simulink model "sliding_quadcopter"  (Simulink 7.9)
settings: Solver=ode4  StartTime=0.0  StopTime=t_end  FixedStep=.01  RelTol=1e-3
values from neighbouring files (symbols this model uses):
  C = [0 0 0]    [gen_smc_starter.m]    (also in pid_starter.m; sliding_starter.m)
  CC_nom = diag([C_nom,Cd_nom])    [gen_smc_starter.m]    (also in sliding_starter.m)
  Cd = [0 0 0]    [gen_smc_starter.m]    (also in pid_starter.m; sliding_starter.m)
  eta = [1 1 1 1]'    [gen_smc_starter.m]    (also in sliding_starter.m = [1 1 1 1 1 1]')
  g = 9.81    [gen_smc_starter.m]    (also in pid_starter.m; sliding_starter.m)
  H_nom = diag([m_nom,m_nom,m_nom,Ix_nom,Iy_nom,Iz_nom])    [gen_smc_starter.m]    (also in sliding_starter.m)
  I = [Ix Iy Iz]    [gen_smc_starter.m]    (also in pid_starter.m; sliding_starter.m)
  Kf = 100    [gen_smc_starter.m]    (also in pid_starter.m; sliding_starter.m)
  Km = 1    [gen_smc_starter.m]    (also in pid_starter.m; sliding_starter.m)
  l = .25    (= 0.25)    [gen_smc_starter.m]    (also in pid_starter.m; sliding_starter.m)
  lamb = [1 20 20 1]    [gen_smc_starter.m]    (also in sliding_starter.m = [5 100 5 .1 .1 .1])
  m = .5    (= 0.5)    [gen_smc_starter.m]    (also in pid_starter.m; sliding_starter.m)
  PSI = [.01 .0005 .0005 .001]'    [gen_smc_starter.m]    (also in sliding_starter.m = [.005 .005 .005 .005 .005 .005]')
  ref = [.1 0 .2 0 0 0]    [gen_smc_starter.m]    (also in pid_starter.m = [.1 -.1 .5 0 0 0]; sliding_starter.m = [0 2 1 0 0 0])
  step_time = [0 0 0]    [gen_smc_starter.m]    (also in pid_starter.m; sliding_starter.m)
  x0 = [0 0        0 0        .2 0        0 0        0 0        0 0        ]    [gen_smc_starter.m]    (also in pid_starter.m = [0 0        0 0        .1 0        0 0        0 0        0 0; sliding_starter.m = [0 0        0 0        .1 0        0 0        0 0        0 0)
settings Model: Creator=dwai  LastModifiedBy=dwai
settings DataIOCC: LimitDataPoints=off
settings DebuggingCC: AlgebraicLoopMsg=none

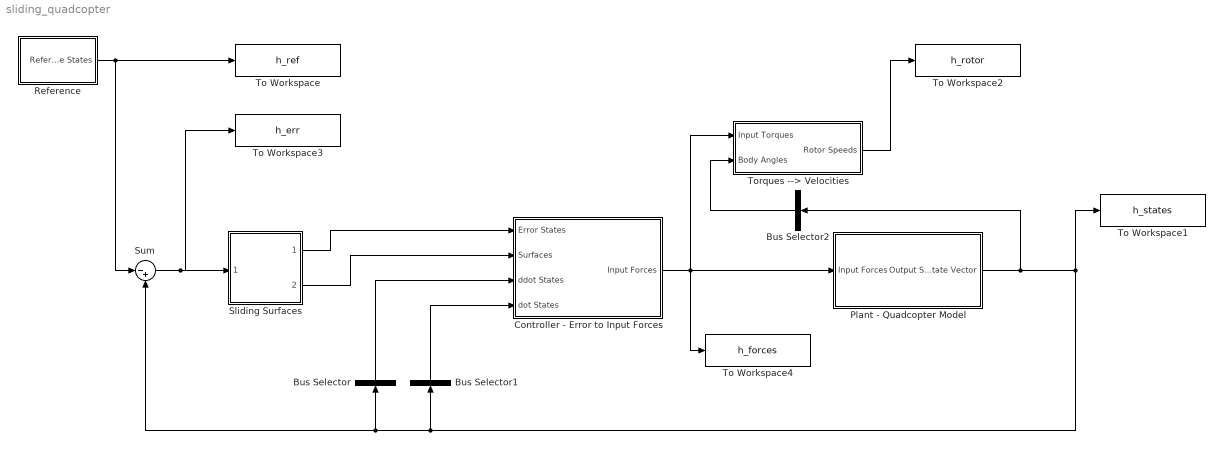
== system sliding_quadcopter ==
  Bus Selector : BusSelector  OutputSignals=x ddot,y ddot,z ddot,phi ddot,th ddot,psi ddot  OutputAsBus=on
  Bus Selector1 : BusSelector  OutputSignals=x dot,y dot,z dot,phi dot,th dot,psi dot  OutputAsBus=on
  Bus Selector2 : BusSelector  OutputSignals=phi,th,psi  OutputAsBus=on
  Controller - Error to Input Forces : Subsystem
  Plant - Quadcopter Model : Subsystem
  Reference : Subsystem
  Sliding Surfaces : Subsystem
  Sum : Sum  Inputs=|-+
  To Workspace : ToWorkspace  VariableName=h_ref  SampleTime=-1  SaveFormat=Timeseries
  To Workspace1 : ToWorkspace  VariableName=h_states  SampleTime=-1  SaveFormat=Timeseries
  To Workspace2 : ToWorkspace  VariableName=h_rotor  SampleTime=-1  SaveFormat=Timeseries
  To Workspace3 : ToWorkspace  VariableName=h_err  SampleTime=-1  SaveFormat=Timeseries
  To Workspace4 : ToWorkspace  VariableName=h_forces  SampleTime=-1  SaveFormat=Timeseries
  Torques --> Velocities : Subsystem
  wires:
  Plant - Quadcopter Model/1(Output State Vector) -> To Workspace1/1, Sum/2, Bus Selector/1, Bus Selector1/1, Bus Selector2/1
  Reference/1(Reference States) -> To Workspace/1, Sum/1
  Sum/1 -> To Workspace3/1, Sliding Surfaces/1(Error States)
  Sliding Surfaces/1(Err States) -> Controller - Error to Input Forces/1(Error States)
  Sliding Surfaces/2(Surfaces) -> Controller - Error to Input Forces/2(Surfaces)
  Bus Selector/1 -> Controller - Error to Input Forces/3(ddot States)
  Bus Selector1/1 -> Controller - Error to Input Forces/4(dot States)
  Controller - Error to Input Forces/1(Input Forces) -> Plant - Quadcopter Model/1(Input Forces), Torques --> Velocities/1(Input Torques), To Workspace4/1
  Torques --> Velocities/1(Rotor Speeds) -> To Workspace2/1
  Bus Selector2/1 -> Torques --> Velocities/2(Body Angles)

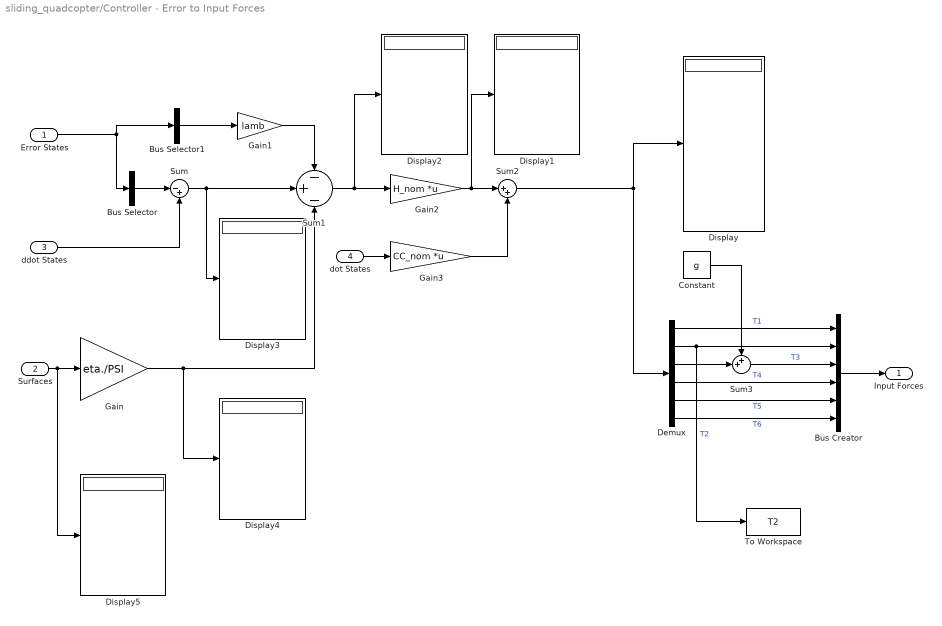
== system sliding_quadcopter/Controller - Error to Input Forces ==
  Error States : Inport
  Surfaces : Inport  Port=2
  ddot States : Inport  Port=3
  dot States : Inport  Port=4
  Bus Creator : BusCreator  Inputs=6
  Bus Selector : BusSelector  OutputSignals=xddot_err,yddot_err,zddot_err,phiddot_err,thddot_err,psiddot_err  OutputAsBus=on
  Bus Selector1 : BusSelector  OutputSignals=xdot_err,ydot_err,zdot_err,phidot_err,thdot_err,psidot_err  OutputAsBus=on
  Constant : Constant  Value=g
  Demux : Demux  Outputs=6
  Display{,1..5} (6 alike) : Display
  Gain : Gain  Gain=eta./PSI
  Gain1 : Gain  Gain=lamb
  Gain2 : Gain  Gain=H_nom  Multiplication=Matrix(K*u)
  Gain3 : Gain  Gain=CC_nom  Multiplication=Matrix(K*u)
  Sum : Sum  Inputs=|-+
  Sum1 : Sum  Inputs=-+-
  Sum2 : Sum  Inputs=|++
  Sum3 : Sum  Inputs=++|
  To Workspace : ToWorkspace  VariableName=T2  SampleTime=-1  SaveFormat=Timeseries
  Input Forces : Outport
  wires:
  Error States/1 -> Bus Selector/1, Bus Selector1/1
  Bus Creator/1 -> Input Forces/1
  Surfaces/1 -> Gain/1, Display5/1
  ddot States/1 -> Sum/2
  Bus Selector/1 -> Sum/1
  Bus Selector1/1 -> Gain1/1
  Gain/1 -> Sum1/3, Display4/1
  Sum/1 -> Sum1/2, Display3/1
  Gain1/1 -> Sum1/1
  dot States/1 -> Gain3/1
  Sum1/1 -> Gain2/1, Display2/1
  Gain2/1 -> Sum2/1, Display1/1
  Gain3/1 -> Sum2/2
  Sum2/1 -> Demux/1, Display/1
  Demux/1 -> Bus Creator/1  "T1"
  Demux/2 -> Bus Creator/2, To Workspace/1  "T2"
  Demux/4 -> Bus Creator/4  "T4"
  Demux/3 -> Sum3/2
  Sum3/1 -> Bus Creator/3  "T3"
  Constant/1 -> Sum3/1
  Demux/5 -> Bus Creator/5  "T5"
  Demux/6 -> Bus Creator/6  "T6"

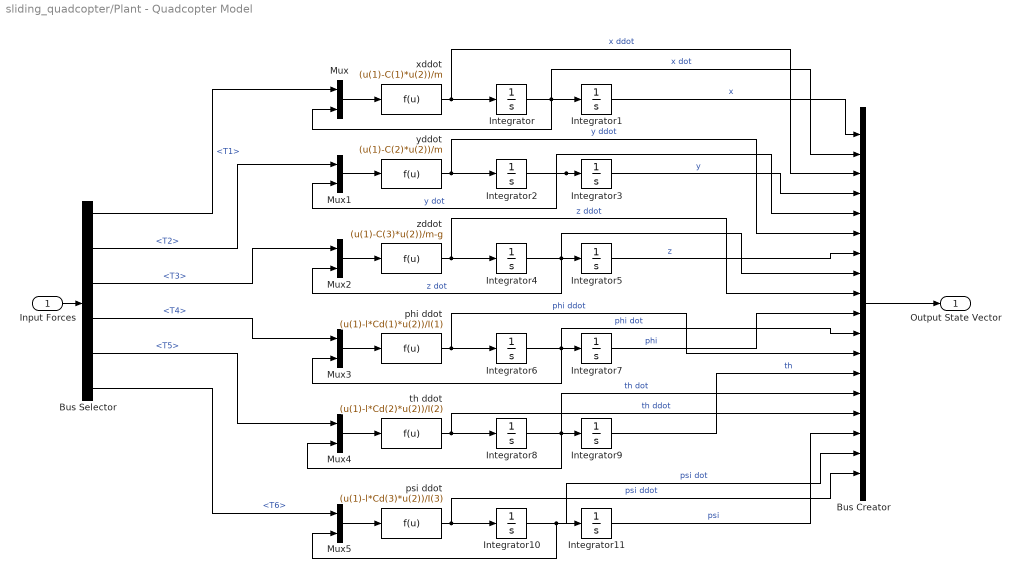
== system sliding_quadcopter/Plant - Quadcopter Model ==
  Input Forces : Inport
  Bus Creator : BusCreator  Inputs=18
  Bus Selector : BusSelector  OutputSignals=T1,T2,T3,T4,T5,T6
  Integrator : Integrator  InitialCondition=x0(2)
  Integrator1 : Integrator  InitialCondition=x0(1)
  Integrator10 : Integrator  InitialCondition=x0(12)
  Integrator11 : Integrator  InitialCondition=x0(11)
  Integrator2 : Integrator  InitialCondition=x0(4)
  Integrator3 : Integrator  InitialCondition=x0(3)
  Integrator4 : Integrator  InitialCondition=x0(6)
  Integrator5 : Integrator  InitialCondition=x0(5)
  Integrator6 : Integrator  InitialCondition=x0(8)
  Integrator7 : Integrator  InitialCondition=x0(7)
  Integrator8 : Integrator  InitialCondition=x0(10)
  Integrator9 : Integrator  InitialCondition=x0(9)
  Mux{,1..5} (6 alike) : Mux  Inputs=2
  phi ddot : Fcn  Expr=(u(1)-l*Cd(1)*u(2))/I(1)
  psi ddot : Fcn  Expr=(u(1)-l*Cd(3)*u(2))/I(3)
  th ddot : Fcn  Expr=(u(1)-l*Cd(2)*u(2))/I(2)
  xddot : Fcn  Expr=(u(1)-C(1)*u(2))/m
  yddot : Fcn  Expr=(u(1)-C(2)*u(2))/m
  zddot : Fcn  Expr=(u(1)-C(3)*u(2))/m-g
  Output State Vector : Outport
  wires:
  Bus Selector/6 -> Mux5/1  "<T6>"
  Bus Selector/5 -> Mux4/1  "<T5>"
  Bus Selector/4 -> Mux3/1  "<T4>"
  Bus Selector/3 -> Mux2/1  "<T3>"
  Bus Selector/2 -> Mux1/1  "<T2>"
  Bus Selector/1 -> Mux/1  "<T1>"
  Integrator11/1 -> Bus Creator/16  "psi"
  Integrator9/1 -> Bus Creator/13  "th"
  Integrator7/1 -> Bus Creator/10  "phi"
  Integrator5/1 -> Bus Creator/7  "z"
  Integrator3/1 -> Bus Creator/4  "y"
  Integrator1/1 -> Bus Creator/1  "x"
  Integrator10/1 -> Integrator11/1, Mux5/2, Bus Creator/17  "psi dot"
  psi ddot/1 -> Integrator10/1, Bus Creator/18  "psi ddot"
  Mux5/1 -> psi ddot/1
  Integrator8/1 -> Integrator9/1, Mux4/2, Bus Creator/14  "th dot"
  th ddot/1 -> Integrator8/1, Bus Creator/15  "th ddot"
  Mux4/1 -> th ddot/1
  Integrator6/1 -> Integrator7/1, Mux3/2, Bus Creator/11  "phi dot"
  phi ddot/1 -> Integrator6/1, Bus Creator/12  "phi ddot"
  Mux3/1 -> phi ddot/1
  Integrator4/1 -> Integrator5/1, Mux2/2, Bus Creator/8  "z dot"
  zddot/1 -> Integrator4/1, Bus Creator/9  "z ddot"
  Mux2/1 -> zddot/1
  Integrator2/1 -> Integrator3/1, Mux1/2, Bus Creator/5  "y dot"
  yddot/1 -> Integrator2/1, Bus Creator/6  "y ddot"
  Mux1/1 -> yddot/1
  Integrator/1 -> Integrator1/1, Mux/2, Bus Creator/2  "x dot"
  xddot/1 -> Integrator/1, Bus Creator/3  "x ddot"
  Mux/1 -> xddot/1
  Bus Creator/1 -> Output State Vector/1
  Input Forces/1 -> Bus Selector/1

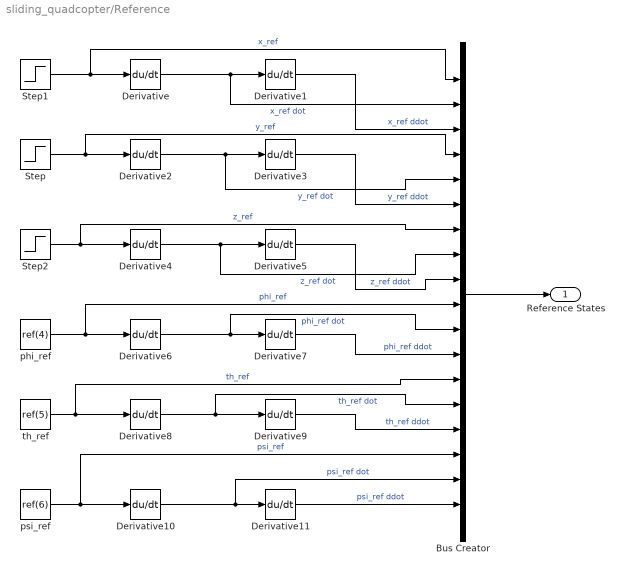
== system sliding_quadcopter/Reference ==
  Bus Creator : BusCreator  Inputs=18
  Derivative{,1..11} (12 alike) : Derivative
  Step : Step  Time=step_time(2)  After=ref(2)  SampleTime=0
  Step1 : Step  Time=step_time(1)  After=ref(1)  SampleTime=0
  Step2 : Step  Time=step_time(3)  After=ref(3)  SampleTime=0
  phi_ref : Constant  Value=ref(4)
  psi_ref : Constant  Value=ref(6)
  th_ref : Constant  Value=ref(5)
  Reference States : Outport
  wires:
  Derivative/1 -> Derivative1/1, Bus Creator/2  "x_ref dot"
  Derivative2/1 -> Derivative3/1, Bus Creator/5  "y_ref dot"
  Step2/1 -> Derivative4/1, Bus Creator/7  "z_ref"
  Derivative4/1 -> Derivative5/1, Bus Creator/8  "z_ref dot"
  phi_ref/1 -> Derivative6/1, Bus Creator/10  "phi_ref"
  Derivative6/1 -> Derivative7/1, Bus Creator/11  "phi_ref dot"
  th_ref/1 -> Derivative8/1, Bus Creator/13  "th_ref"
  Derivative8/1 -> Derivative9/1, Bus Creator/14  "th_ref dot"
  psi_ref/1 -> Derivative10/1, Bus Creator/16  "psi_ref"
  Derivative10/1 -> Derivative11/1, Bus Creator/17  "psi_ref dot"
  Derivative1/1 -> Bus Creator/3  "x_ref ddot"
  Derivative3/1 -> Bus Creator/6  "y_ref ddot"
  Derivative5/1 -> Bus Creator/9  "z_ref ddot"
  Derivative7/1 -> Bus Creator/12  "phi_ref ddot"
  Derivative9/1 -> Bus Creator/15  "th_ref ddot"
  Derivative11/1 -> Bus Creator/18  "psi_ref ddot"
  Bus Creator/1 -> Reference States/1
  Step/1 -> Derivative2/1, Bus Creator/4  "y_ref"
  Step1/1 -> Derivative/1, Bus Creator/1  "x_ref"

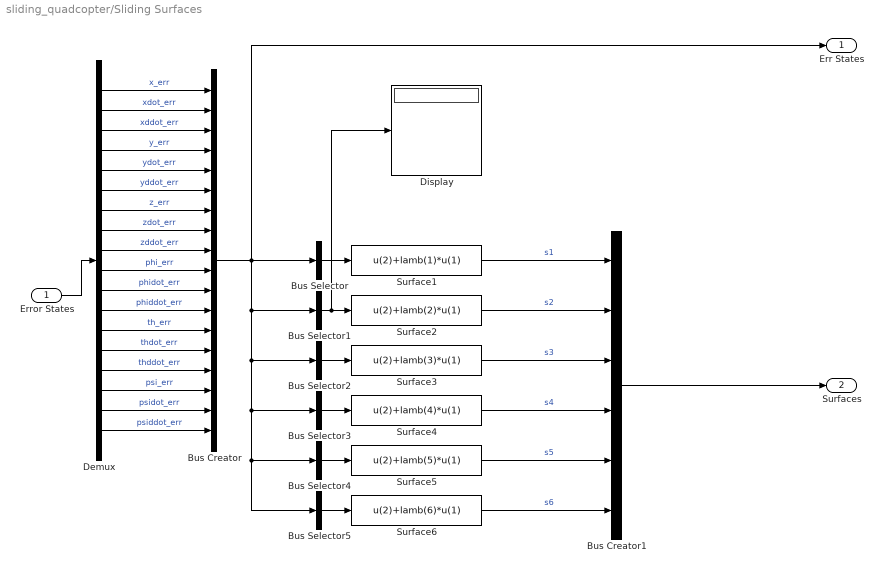
== system sliding_quadcopter/Sliding Surfaces ==
  Error States : Inport
  Bus Creator : BusCreator  Inputs=18
  Bus Creator1 : BusCreator  Inputs=6
  Bus Selector : BusSelector  OutputSignals=x_err,xdot_err  OutputAsBus=on
  Bus Selector1 : BusSelector  OutputSignals=y_err,ydot_err  OutputAsBus=on
  Bus Selector2 : BusSelector  OutputSignals=z_err,zdot_err  OutputAsBus=on
  Bus Selector3 : BusSelector  OutputSignals=phi_err,phidot_err  OutputAsBus=on
  Bus Selector4 : BusSelector  OutputSignals=th_err,thdot_err  OutputAsBus=on
  Bus Selector5 : BusSelector  OutputSignals=psi_err,psidot_err  OutputAsBus=on
  Demux : Demux  Outputs=18
  Display : Display
  Surface1 : Fcn  Expr=u(2)+lamb(1)*u(1)
  Surface2 : Fcn  Expr=u(2)+lamb(2)*u(1)
  Surface3 : Fcn  Expr=u(2)+lamb(3)*u(1)
  Surface4 : Fcn  Expr=u(2)+lamb(4)*u(1)
  Surface5 : Fcn  Expr=u(2)+lamb(5)*u(1)
  Surface6 : Fcn  Expr=u(2)+lamb(6)*u(1)
  Err States : Outport
  Surfaces : Outport  Port=2
  wires:
  Error States/1 -> Demux/1
  Bus Creator/1 -> Err States/1, Bus Selector/1, Bus Selector5/1, Bus Selector4/1, Bus Selector3/1, Bus Selector2/1, Bus Selector1/1
  Bus Creator1/1 -> Surfaces/1
  Demux/18 -> Bus Creator/18  "psiddot_err"
  Demux/17 -> Bus Creator/17  "psidot_err"
  Demux/16 -> Bus Creator/16  "psi_err"
  Demux/15 -> Bus Creator/15  "thddot_err"
  Demux/14 -> Bus Creator/14  "thdot_err"
  Demux/13 -> Bus Creator/13  "th_err"
  Demux/12 -> Bus Creator/12  "phiddot_err"
  Demux/11 -> Bus Creator/11  "phidot_err"
  Demux/10 -> Bus Creator/10  "phi_err"
  Demux/9 -> Bus Creator/9  "zddot_err"
  Demux/8 -> Bus Creator/8  "zdot_err"
  Demux/7 -> Bus Creator/7  "z_err"
  Demux/6 -> Bus Creator/6  "yddot_err"
  Demux/5 -> Bus Creator/5  "ydot_err"
  Demux/4 -> Bus Creator/4  "y_err"
  Demux/3 -> Bus Creator/3  "xddot_err"
  Demux/2 -> Bus Creator/2  "xdot_err"
  Demux/1 -> Bus Creator/1  "x_err"
  Bus Selector/1 -> Surface1/1
  Bus Selector1/1 -> Surface2/1, Display/1
  Bus Selector2/1 -> Surface3/1
  Bus Selector3/1 -> Surface4/1
  Bus Selector4/1 -> Surface5/1
  Bus Selector5/1 -> Surface6/1
  Surface1/1 -> Bus Creator1/1  "s1"
  Surface2/1 -> Bus Creator1/2  "s2"
  Surface3/1 -> Bus Creator1/3  "s3"
  Surface4/1 -> Bus Creator1/4  "s4"
  Surface5/1 -> Bus Creator1/5  "s5"
  Surface6/1 -> Bus Creator1/6  "s6"

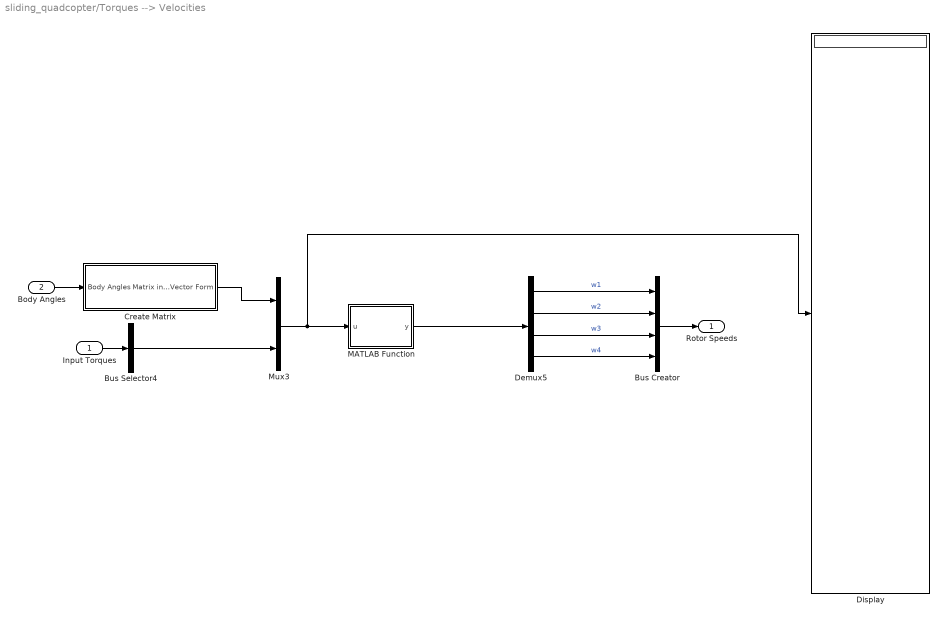
== system sliding_quadcopter/Torques --> Velocities ==
  Input Torques : Inport
  Body Angles : Inport  Port=2
  Bus Creator : BusCreator
  Bus Selector4 : BusSelector  OutputSignals=T1,T2,T3,T4,T5,T6  OutputAsBus=on
  Create Matrix : Subsystem
  Demux5 : Demux
  Display : Display
  MATLAB Function : MATLAB Function  TreatAsAtomicUnit=on
  Mux3 : Mux  Inputs=2
  Rotor Speeds : Outport
  wires:
  Input Torques/1 -> Bus Selector4/1
  Bus Creator/1 -> Rotor Speeds/1
  Demux5/1 -> Bus Creator/1  "w1"
  Demux5/2 -> Bus Creator/2  "w2"
  Demux5/3 -> Bus Creator/3  "w3"
  Demux5/4 -> Bus Creator/4  "w4"
  MATLAB Function/1(y) -> Demux5/1
  Bus Selector4/1 -> Mux3/2
  Mux3/1 -> MATLAB Function/1(u), Display/1
  Body Angles/1 -> Create Matrix/1(Body Angles)
  Create Matrix/1(Matrix in Vector Form) -> Mux3/1

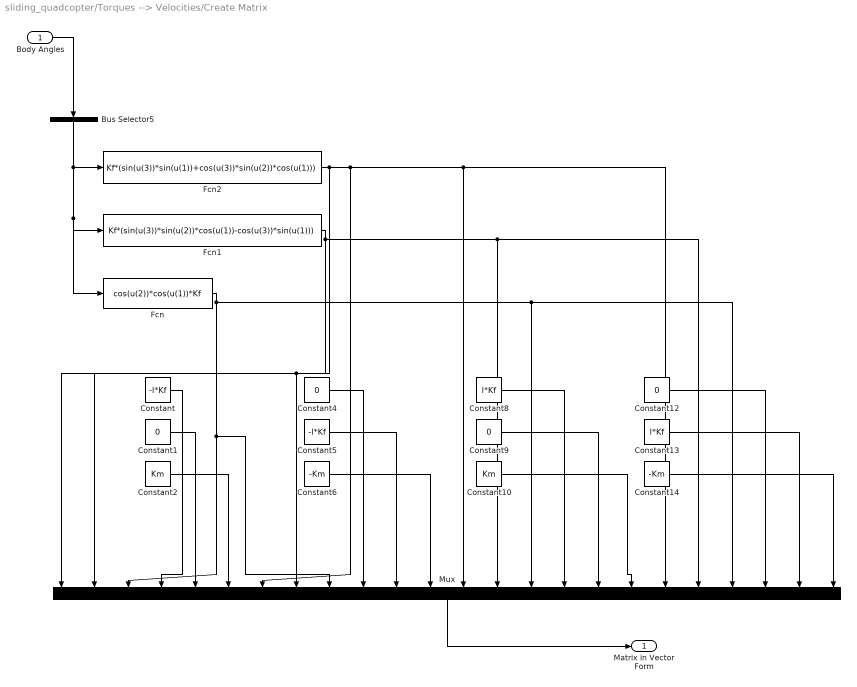
== system sliding_quadcopter/Torques --> Velocities/Create Matrix ==
  Body Angles : Inport
  Bus Selector5 : BusSelector  OutputSignals=phi,th,psi  OutputAsBus=on
  Constant : Constant  Value=-l*Kf
  Constant{1,4,9,12} (4 alike) : Constant  Value=0
  Constant10 : Constant  Value=Km
  Constant13 : Constant  Value=l*Kf
  Constant14 : Constant  Value=-Km
  Constant2 : Constant  Value=Km
  Constant5 : Constant  Value=-l*Kf
  Constant6 : Constant  Value=-Km
  Constant8 : Constant  Value=l*Kf
  Fcn : Fcn  Expr=cos(u(2))*cos(u(1))*Kf
  Fcn1 : Fcn  Expr=Kf*(sin(u(3))*sin(u(2))*cos(u(1))-cos(u(3))*sin(u(1)))
  Fcn2 : Fcn  Expr=Kf*(sin(u(3))*sin(u(1))+cos(u(3))*sin(u(2))*cos(u(1)))
  Mux : Mux  Inputs=24
  Matrix in Vector Form : Outport
  wires:
  Body Angles/1 -> Bus Selector5/1
  Mux/1 -> Matrix in Vector Form/1
  Bus Selector5/1 -> Fcn2/1, Fcn1/1, Fcn/1
  Fcn2/1 -> Mux/1, Mux/7, Mux/13, Mux/19
  Fcn1/1 -> Mux/2, Mux/8, Mux/14, Mux/20
  Fcn/1 -> Mux/3, Mux/9, Mux/15, Mux/21
  Constant/1 -> Mux/4
  Constant1/1 -> Mux/5
  Constant2/1 -> Mux/6
  Constant4/1 -> Mux/10
  Constant5/1 -> Mux/11
  Constant6/1 -> Mux/12
  Constant8/1 -> Mux/16
  Constant9/1 -> Mux/17
  Constant10/1 -> Mux/18
  Constant12/1 -> Mux/22
  Constant13/1 -> Mux/23
  Constant14/1 -> Mux/24

== matlab function Torques --> Velocities/MATLAB Function ==
  data: u input double; y output double
function y = fcn(u)

vector = u(1:24);
torques = u(25:30);
A = reshape(vector,6,4)
y = A\torques;
